simulink model "part_MAIN"  (R2023b)
settings: Solver=ode4  StartTime=0.0  StopTime=2000  FixedStep=0.1  RelTol=1e-3
values from neighbouring files (symbols this model uses):
  Af = diag(ti)    [init.m]
  change_position_time = 400    [init.m]
  Gamma = diag(omega_is)    [init.m]
  Kd = [1660451.40544401; 3920391.80535684; 1605063439.04156]    [init.m]
  Ki = [137.081306245593; 763.274947400198; 335358.448218978]    [init.m]
  Kp = [75459.3345349083; 277551.73586971; 120744473.878042]    [init.m]
  Omega = diag(2*omega_is.*zeta_is)    [init.m]
  simulation = 4    [init.m]
undefined symbols (not defined in the file or in its folder): Hoerner, vessel
libraries: simulink x2, marine_hydro x1
settings Model: Creator=jonbjor  LastModifiedBy=aduragbemi
settings SolverCC: AlgebraicLoopSolver=TrustRegion
settings DataIOCC: ReturnWorkspaceOutputs=off
settings DebuggingCC: UnconnectedInputMsg=warning  UnconnectedOutputMsg=warning  UnconnectedLineMsg=warning  ArithmeticOperatorsInVariantConditions=warning
settings ModelReferenceCC: EnableRefExpFcnMdlSchedulingChecks=on
settings SFSimCC: SimUseLocalCustomCode=off  CustomCodeUndefinedFunction=UseInterfaceOnly
settings RTWCC: RTWUseLocalCustomCode=off  DLArmComputeVersion=19.05

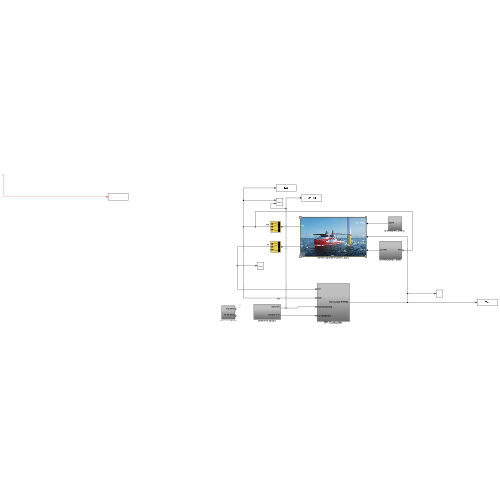
[thumbnail: Simulink's stored preview of the top-level diagram]
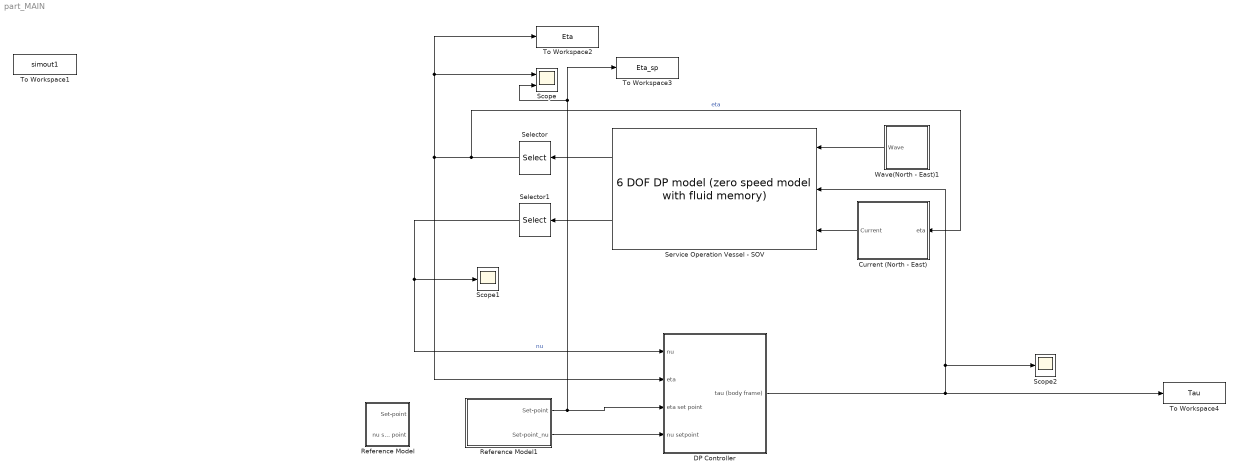
== system part_MAIN ==
  Current (North - East) : Subsystem
  DP Controller : Subsystem
  Reference Model : Subsystem
  Reference Model1 : Subsystem
  Scope : Scope  NumInputPorts=2
  Scope1 : Scope
  Scope2 : Scope
  Selector : Selector  InputPortWidth=6  IndexOptions=Index vector (dialog)  Indices=[1 2 6]  OutputSizes=1
  Selector1 : Selector  InputPortWidth=6  IndexOptions=Index vector (dialog)  Indices=[1 2 6]  OutputSizes=1
  Service Operation Vessel - SOV : marine_hydro/Hydro Library/6 DOF DP model  (zero speed model with fluid memory)  ABC=vesselABC  rho=1025  Axc=0.9*vessel.main.T*vessel.main.B  Ayc=0.9*vessel.main.T*vessel.main.Lpp  CX=1  CY_2D=Hoerner(vessel.main.B,vessel.main.T)  Bv=vessel.Bv  mask(6 DOF zero speed model){}
      link override "Integrator1 ": InitialCondition=nu0
      link override Integrator2: InitialCondition=eta0
      mask Display:
      | image('SOV.jpg');
      | color('white'); port_label('output', 1, 'eta')
      | color('white'); port_label('output', 2, 'nu')
      | color('white'); port_label('input', 1, 'tau_wave')
      | color('white'); port_label('input', 2, 'tau')
      | color('white'); port_label('input', 3, 'nu_c')
  To Workspace1 : ToWorkspace  VariableName=simout1  SaveFormat=Timeseries  SampleTime=-1
  To Workspace2 : ToWorkspace  VariableName=Eta  SaveFormat=Timeseries  SampleTime=-1
  To Workspace3 : ToWorkspace  VariableName=Eta_sp  SaveFormat=Timeseries  SampleTime=-1
  To Workspace4 : ToWorkspace  VariableName=Tau  SaveFormat=Timeseries  SampleTime=-1
  Wave(North - East)1 : Subsystem
  wires:
  Current (North - East)/1(Current) -> Service Operation Vessel - SOV/3
  DP Controller/1(tau (body frame)) -> Scope2/1, Service Operation Vessel - SOV/2, To Workspace4/1
  Service Operation Vessel - SOV/1 -> Selector/1
  Service Operation Vessel - SOV/2 -> Selector1/1
  Selector/1 -> Current (North - East)/1(eta), To Workspace2/1, Scope/1, DP Controller/2(eta)  "eta"
  Selector1/1 -> Scope1/1, DP Controller/1(nu)  "nu"
  Wave(North - East)1/1(Wave) -> Service Operation Vessel - SOV/1
  Reference Model1/2(Set-point_nu) -> DP Controller/4(nu setpoint)
  ? -> To Workspace1/1
  Reference Model1/1(Set-point) -> Scope/2, To Workspace3/1, DP Controller/3(eta set point)

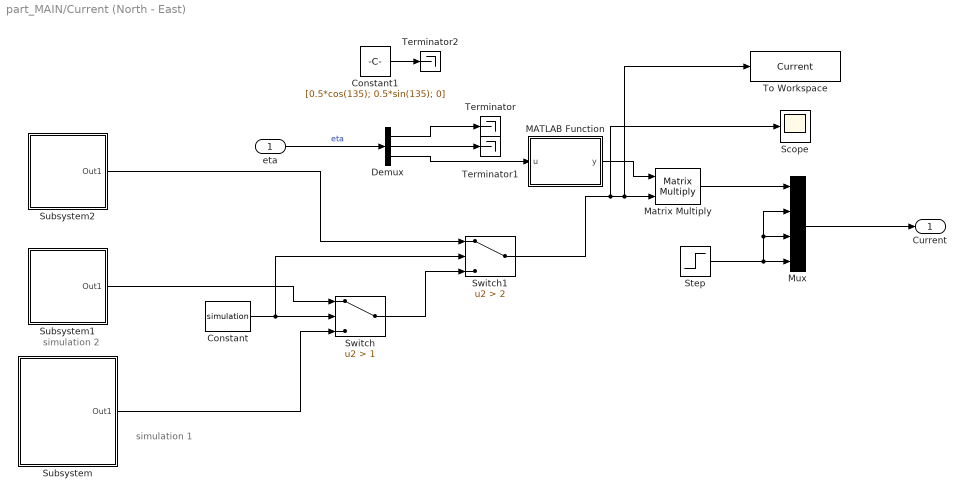
== system part_MAIN/Current (North - East) ==
  note: simulation 2
  note: simulation 1
  eta : Inport
  Constant : Constant  Value=simulation
  Constant1 : Constant  Value=[0.5*cos(135); 0.5*sin(135); 0]
  Demux : Demux  Outputs=3
  MATLAB Function : MATLAB Function  TreatAsAtomicUnit=on
  Matrix Multiply : Product  Multiplication=Matrix(*)
  Mux : Mux
  Scope : Scope
  Step : Step  After=0  SampleTime=0
  Subsystem : Subsystem
  Subsystem1 : Subsystem
  Subsystem2 : Subsystem
  Switch : Switch  Criteria=u2 > Threshold  Threshold=1  SaturateOnIntegerOverflow=off  InputSameDT=off
  Switch1 : Switch  Criteria=u2 > Threshold  Threshold=2  SaturateOnIntegerOverflow=off  InputSameDT=off
  Terminator : Terminator
  Terminator1 : Terminator
  Terminator2 : Terminator
  To Workspace : ToWorkspace  VariableName=Current  SaveFormat=Timeseries  SampleTime=-1
  Current : Outport  VectorParamsAs1DForOutWhenUnconnected=off
  wires:
  Demux/1 -> Terminator/1
  Demux/2 -> Terminator1/1
  Demux/3 -> MATLAB Function/1(u)
  MATLAB Function/1(y) -> Matrix Multiply/1
  Mux/1 -> Current/1
  Matrix Multiply/1 -> Mux/1
  Step/1 -> Mux/3, Mux/2, Mux/4
  eta/1 -> Demux/1  "eta"
  Constant1/1 -> Terminator2/1
  Subsystem/1(Out1) -> Switch/3
  Constant/1 -> Switch1/2, Switch/2
  Subsystem1/1(Out1) -> Switch/1
  Switch/1 -> Switch1/3
  Subsystem2/1(Out1) -> Switch1/1
  Switch1/1 -> Scope/1, To Workspace/1, Matrix Multiply/2

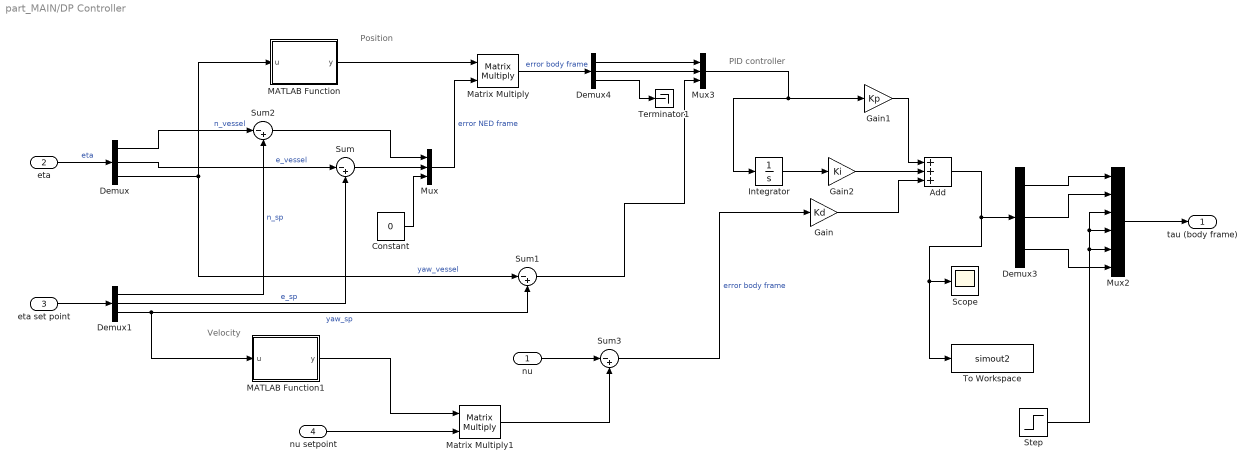
== system part_MAIN/DP Controller ==
  note: PID controller
  note: Velocity
  note: Position
  nu : Inport
  eta : Inport  Port=2
  eta set point : Inport  Port=3
  nu setpoint : Inport  Port=4
  Add : Sum  Inputs=+++
  Constant : Constant  Value=0
  Demux{,1,3..4} (4 alike) : Demux  Outputs=3
  Gain : Gain  Gain=Kd
  Gain1 : Gain  Gain=Kp
  Gain2 : Gain  Gain=Ki
  Integrator : Integrator
  MATLAB Function : MATLAB Function  TreatAsAtomicUnit=on
  MATLAB Function1 : MATLAB Function  TreatAsAtomicUnit=on
  Matrix Multiply : Product  Multiplication=Matrix(*)
  Matrix Multiply1 : Product  Multiplication=Matrix(*)
  Mux : Mux  Inputs=3
  Mux2 : Mux  Inputs=6
  Mux3 : Mux  Inputs=3
  Scope : Scope
  Step : Step  After=0  SampleTime=0
  Sum{,1..3} (4 alike) : Sum  Inputs=|-+
  Terminator1 : Terminator
  To Workspace : ToWorkspace  VariableName=simout2  SaveFormat=Timeseries  SampleTime=-1
  tau (body frame) : Outport  VectorParamsAs1DForOutWhenUnconnected=off
  wires:
  eta/1 -> Demux/1  "eta"
  eta set point/1 -> Demux1/1
  Demux/1 -> Sum2/1  "n_vessel"
  Demux1/1 -> Sum2/2  "n_sp"
  Demux/2 -> Sum/1  "e_vessel"
  Demux1/2 -> Sum/2  "e_sp"
  Sum2/1 -> Mux/1
  Sum/1 -> Mux/2
  MATLAB Function/1(y) -> Matrix Multiply/1
  Mux/1 -> Matrix Multiply/2  "error NED frame"
  Step/1 -> Mux2/4, Mux2/3, Mux2/5
  Demux1/3 -> MATLAB Function1/1(u), Sum1/2  "yaw_sp"
  Sum1/1 -> Mux3/3
  Constant/1 -> Mux/3
  Demux/3 -> MATLAB Function/1(u), Sum1/1  "yaw_vessel"
  Matrix Multiply/1 -> Demux4/1  "error body frame"
  nu/1 -> Sum3/1
  Sum3/1 -> Gain/1  "error body frame"
  nu setpoint/1 -> Matrix Multiply1/2
  MATLAB Function1/1(y) -> Matrix Multiply1/1
  Matrix Multiply1/1 -> Sum3/2
  Integrator/1 -> Gain2/1
  Gain1/1 -> Add/1
  Gain2/1 -> Add/2
  Gain/1 -> Add/3
  Add/1 -> To Workspace/1, Scope/1, Demux3/1
  Demux3/1 -> Mux2/1
  Demux3/2 -> Mux2/2
  Demux3/3 -> Mux2/6
  Mux2/1 -> tau (body frame)/1
  Demux4/1 -> Mux3/1
  Demux4/2 -> Mux3/2
  Demux4/3 -> Terminator1/1
  Mux3/1 -> Integrator/1, Gain1/1

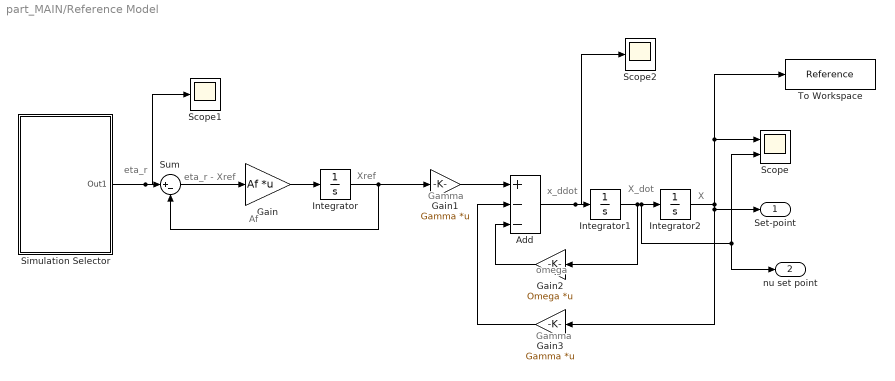
== system part_MAIN/Reference Model ==
  note: Af
  note: eta_r
  note: Xref
  note: omega
  note: eta_r - Xref
  note: Gamma
  note: x_ddot
  note: Gamma
  note: X_dot
  note: X
  Add : Sum  Inputs=+--
  Gain : Gain  Gain=Af  Multiplication=Matrix(K*u)
  Gain1 : Gain  Gain=Gamma  Multiplication=Matrix(K*u)
  Gain2 : Gain  Gain=Omega  Multiplication=Matrix(K*u)
  Gain3 : Gain  Gain=Gamma  Multiplication=Matrix(K*u)
  Integrator : Integrator
  Integrator1 : Integrator
  Integrator2 : Integrator
  Scope : Scope  NumInputPorts=2
  Scope1 : Scope
  Scope2 : Scope
  Simulation Selector : Subsystem
  Sum : Sum  Inputs=|+-
  To Workspace : ToWorkspace  VariableName=Reference  SaveFormat=Timeseries  SampleTime=-1
  Set-point : Outport  VectorParamsAs1DForOutWhenUnconnected=off
  nu set point : Outport  Port=2  VectorParamsAs1DForOutWhenUnconnected=off
  wires:
  Integrator/1 -> Gain1/1, Sum/2
  Add/1 -> Scope2/1, Integrator1/1
  Integrator2/1 -> To Workspace/1, Scope/1, Set-point/1, Gain3/1
  Gain1/1 -> Add/1
  Integrator1/1 -> nu set point/1, Scope/2, Integrator2/1, Gain2/1
  Gain/1 -> Integrator/1
  Gain2/1 -> Add/3
  Gain3/1 -> Add/2
  Simulation Selector/1(Out1) -> Scope1/1, Sum/1
  Sum/1 -> Gain/1

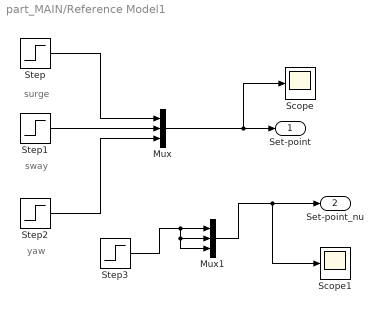
== system part_MAIN/Reference Model1 ==
  note: sway
  note: surge
  note: yaw
  Mux : Mux  Inputs=3
  Mux1 : Mux  Inputs=3
  Scope : Scope
  Scope1 : Scope
  Step : Step  After=10  SampleTime=0
  Step1 : Step  After=10  SampleTime=0
  Step2 : Step  After=3*pi/2  SampleTime=0
  Step3 : Step  After=0  SampleTime=0
  Set-point : Outport
  Set-point_nu : Outport  Port=2
  wires:
  Step2/1 -> Mux/3
  Mux/1 -> Scope/1, Set-point/1
  Step/1 -> Mux/1
  Step1/1 -> Mux/2
  Step3/1 -> Mux1/3, Mux1/2, Mux1/1
  Mux1/1 -> Scope1/1, Set-point_nu/1

== system part_MAIN/Wave(North - East)1 ==
  Constant : Constant  Value=[0; 0; 0; 0; 0; 0]
  Wave : Outport  VectorParamsAs1DForOutWhenUnconnected=off
  wires:
  Constant/1 -> Wave/1

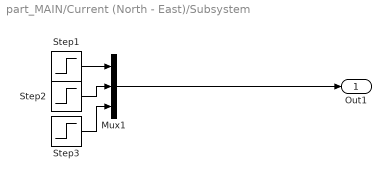
== system part_MAIN/Current (North - East)/Subsystem ==
  Mux1 : Mux  Inputs=3
  Step1 : Step  Time=0  After=0.5*cos(135)  SampleTime=0
  Step2 : Step  Time=0  After=0.5*sin(135)  SampleTime=0
  Step3 : Step  Time=0  After=0  SampleTime=0
  Out1 : Outport
  wires:
  Mux1/1 -> Out1/1
  Step1/1 -> Mux1/1
  Step2/1 -> Mux1/2
  Step3/1 -> Mux1/3

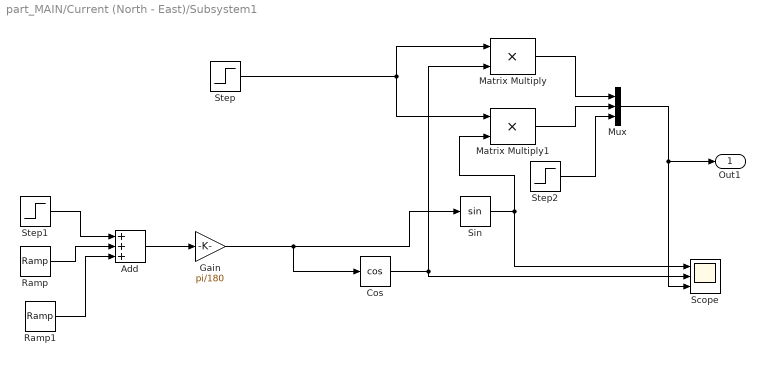
== system part_MAIN/Current (North - East)/Subsystem1 ==
  Add : Sum  Inputs=+++
  Cos : Trigonometry  Operator=cos
  Gain : Gain  Gain=pi/180
  Matrix Multiply : Product
  Matrix Multiply1 : Product
  Mux : Mux  Inputs=3
  Ramp : simulink/Sources/Ramp  slope=0.45  start=2  InitialOutput=0
  Ramp1 : simulink/Sources/Ramp  slope=-0.45  start=202  InitialOutput=0
  Scope : Scope  NumInputPorts=3
  Sin : Trigonometry
  Step : Step  Time=2  After=0.5  SampleTime=0
  Step1 : Step  Time=2  Before=180  After=180  SampleTime=0
  Step2 : Step  Time=0  After=0  SampleTime=0
  Out1 : Outport
  wires:
  Step1/1 -> Add/1
  Ramp/1 -> Add/2
  Ramp1/1 -> Add/3
  Step/1 -> Matrix Multiply1/1, Matrix Multiply/1
  Sin/1 -> Matrix Multiply1/2, Scope/1
  Cos/1 -> Matrix Multiply/2, Scope/2
  Matrix Multiply/1 -> Mux/1
  Matrix Multiply1/1 -> Mux/2
  Step2/1 -> Mux/3
  Mux/1 -> Scope/3, Out1/1
  Add/1 -> Gain/1
  Gain/1 -> Sin/1, Cos/1

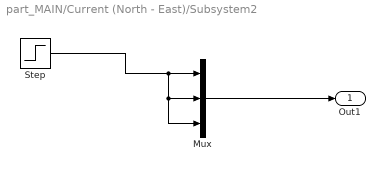
== system part_MAIN/Current (North - East)/Subsystem2 ==
  Mux : Mux  Inputs=3
  Step : Step  Time=0  After=0  SampleTime=0
  Out1 : Outport
  wires:
  Mux/1 -> Out1/1
  Step/1 -> Mux/3, Mux/2, Mux/1

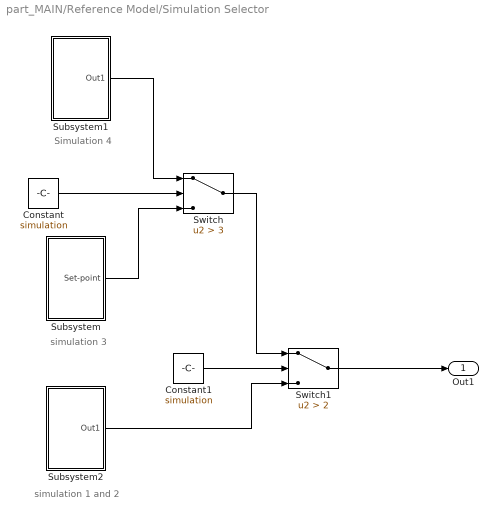
== system part_MAIN/Reference Model/Simulation Selector ==
  note: simulation 1 and 2
  note: Simulation 4
  note: simulation 3
  Constant : Constant  Value=simulation
  Constant1 : Constant  Value=simulation
  Subsystem : Subsystem
  Subsystem1 : Subsystem
  Subsystem2 : Subsystem
  Switch : Switch  Criteria=u2 > Threshold  Threshold=3  SaturateOnIntegerOverflow=off  InputSameDT=off
  Switch1 : Switch  Criteria=u2 > Threshold  Threshold=2  SaturateOnIntegerOverflow=off  InputSameDT=off
  Out1 : Outport
  wires:
  Subsystem1/1(Out1) -> Switch/1
  Subsystem/1(Set-point) -> Switch/3
  Constant/1 -> Switch/2
  Switch/1 -> Switch1/1
  Constant1/1 -> Switch1/2
  Subsystem2/1(Out1) -> Switch1/3
  Switch1/1 -> Out1/1

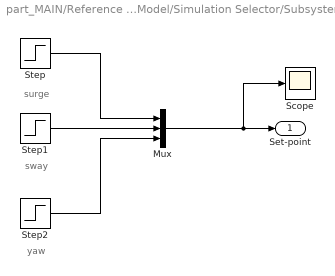
== system part_MAIN/Reference Model/Simulation Selector/Subsystem ==
  note: yaw
  note: sway
  note: surge
  Mux : Mux  Inputs=3
  Scope : Scope
  Step : Step  After=10  SampleTime=0
  Step1 : Step  After=10  SampleTime=0
  Step2 : Step  After=3*pi/2  SampleTime=0
  Set-point : Outport
  wires:
  Step/1 -> Mux/1
  Step1/1 -> Mux/2
  Step2/1 -> Mux/3
  Mux/1 -> Scope/1, Set-point/1

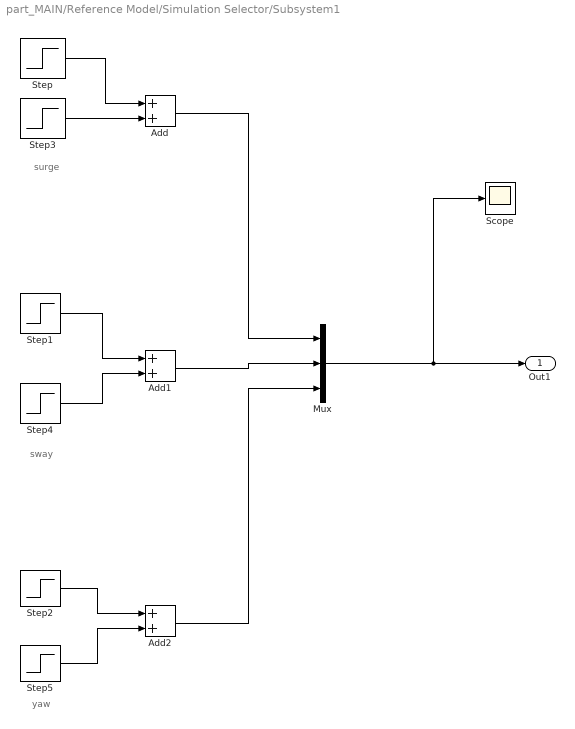
== system part_MAIN/Reference Model/Simulation Selector/Subsystem1 ==
  note: yaw
  note: sway
  note: surge
  Add : Sum
  Add1 : Sum
  Add2 : Sum
  Mux : Mux  Inputs=3
  Scope : Scope
  Step : Step  Time=10  After=50  SampleTime=0
  Step1 : Step  Time=change_position_time  After=-50  SampleTime=0
  Step2 : Step  Time=change_position_time*2  After=pi/4  SampleTime=0
  Step3 : Step  Time=change_position_time*3  After=-50  SampleTime=0
  Step4 : Step  Time=change_position_time*4  After=50  SampleTime=0
  Step5 : Step  Time=change_position_time*4  After=-pi/4  SampleTime=0
  Out1 : Outport
  wires:
  Mux/1 -> Scope/1, Out1/1
  Step/1 -> Add/1
  Step3/1 -> Add/2
  Step1/1 -> Add1/1
  Step4/1 -> Add1/2
  Step2/1 -> Add2/1
  Step5/1 -> Add2/2
  Add/1 -> Mux/1
  Add1/1 -> Mux/2
  Add2/1 -> Mux/3

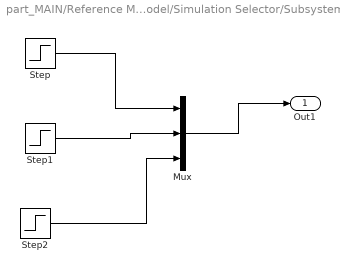
== system part_MAIN/Reference Model/Simulation Selector/Subsystem2 ==
  Mux : Mux  Inputs=3
  Step : Step  After=0  SampleTime=0
  Step1 : Step  After=0  SampleTime=0
  Step2 : Step  After=0  SampleTime=0
  Out1 : Outport
  wires:
  Step/1 -> Mux/1
  Step1/1 -> Mux/2
  Step2/1 -> Mux/3
  Mux/1 -> Out1/1

== matlab function part_MAIN/DP Controller/MATLAB Function ==
  data: u input; y output
function y = fcn(u)

rot = [cos(u) -sin(u) 0;
    sin(u) cos(u) 0;
    0 0 1];

y = rot';

== matlab function part_MAIN/DP Controller/MATLAB Function1 ==
  data: u input; y output
function y = fcn(u)

rot = [cos(u) -sin(u) 0;
    sin(u) cos(u) 0;
    0 0 1];

y = rot';

== matlab function part_MAIN/Current (North - East)/MATLAB Function ==
  data: u input; y output
function y = fcn(u)
rot = [cos(u) -sin(u) 0;
    sin(u) cos(u) 0;
    0 0 1];

y = rot';
